simulink model "GeneralFEVmodel"  (R2022a)
settings: Solver=ode4  StartTime=0  StopTime=endtime  MaxStep=0.05  RelTol=1e-5
values from neighbouring files (symbols this model uses):
  EtaEM = Eta    [CreateEMmapII.m]
  Pbatt_max_new = 150*Mbatt    [CreateBATTmap.m]
  PtoTem = zeros(length(Pem),4)    [CreateEMmapII.m]
  Tem = Tem_max.*Tref/max(Tref)    [CreateEMmapII.m]
  Tem_lim = min([Tem_max*ones(1,length(Wem)); Pem_max./Wem])    [CreateEMmapII.m]
  Wem = wem_max.*w/max(w)    [CreateEMmapII.m]
undefined symbols (not defined in the file or in its folder): Av, Cd, Cr, EtaBATT, EtaGEAR, EtaPE, grav, Mv, Number_of_gears, Paux, Pbatt, Pem_max, rho_air, rw, SOC_batt_start_value, SOC_tract_max, SOC_tract_min, Tem_max, utvx_max, Utvx_vect, Wbatt, wem_max, wem_min
libraries: simulink_need_slupdate x1, simulink x1
settings Model: ExtModeTrigMode=oneshot  ExtModeArmWhenConnect=off  Creator=Mats  LastModifiedBy=Albin
settings SolverCC: AlgebraicLoopSolver=TrustRegion
settings DataIOCC: SaveFormat=Array  SignalLoggingSaveFormat=ModelDataLogs  ReturnWorkspaceOutputs=off  SignalLoggingName=sigsOut
settings OptimizationCC: BlockReduction=off  BooleanDataType=off  DefaultParameterBehavior=Inlined  BufferReuse=off  ExpressionDepthLimit=2147483647  InitFltsAndDblsToZero=on  LifeSpan=inf
settings DebuggingCC: ConsistencyChecking=warning  SaveWithParameterizedLinksMsg=none  UnderspecifiedInitializationDetection=Classic  MergeDetectMultiDrivingBlocksExec=none  SignalResolutionControl=TryResolveAllWithWarning  MultiTaskDSMMsg=warning  MultiTaskCondExecSysMsg=none  UnnecessaryDatatypeConvMsg=warning  FcnCallInpInsideContextMsg=warning  StateNameClashWarn=warning  SFUnexpectedBacktrackingDiag=warning  SFNoUnconditionalDefaultTransitionDiag=warning  SFMachineParentedDataDiag=warning  ArithmeticOperatorsInVariantConditions=warning
settings HardwareCC: ProdBitPerPointer=32  ProdBitPerSizeT=32  ProdBitPerPtrDiffT=32  ProdLargestAtomicFloat=None  ProdIntDivRoundTo=Undefined  ProdEndianess=Unspecified  ProdWordSize=32  ProdHWDeviceType=32-bit Generic  TargetHWDeviceType=32-bit Generic  TargetUnknown=on  ProdEqTarget=off
settings ModelReferenceCC: PropagateSignalLabelsOutOfModel=off
settings SFSimCC: SimUseLocalCustomCode=off  CustomCodeUndefinedFunction=UseInterfaceOnly
settings RTWCC: RTWUseLocalCustomCode=off  DLArmComputeVersion=19.05
settings CodeAppCC: StateflowObjectComments=on
settings GRTTargetCC: TargetFcnLib=ansi_tfl_tmw.mat  TargetLangStandard=C89/C90 (ANSI)  CombineOutputUpdateFcns=off  GRTInterface=on
settings ConfigComp: CovMetricSettings=dw  CovSaveCumulativeToWorkspaceVar=on  CovSaveSingleToWorkspaceVar=on  CovExternalEMLEnable=off

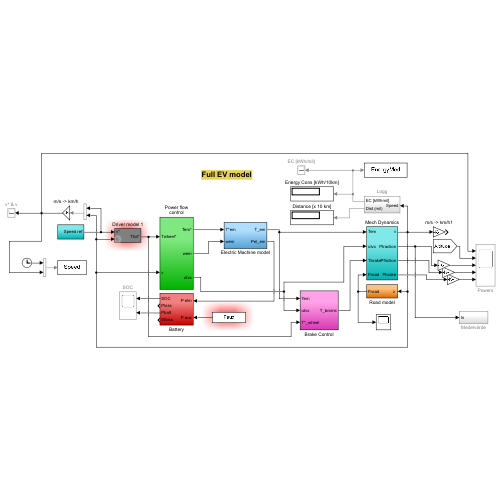
[thumbnail: Simulink's stored preview of the top-level diagram]
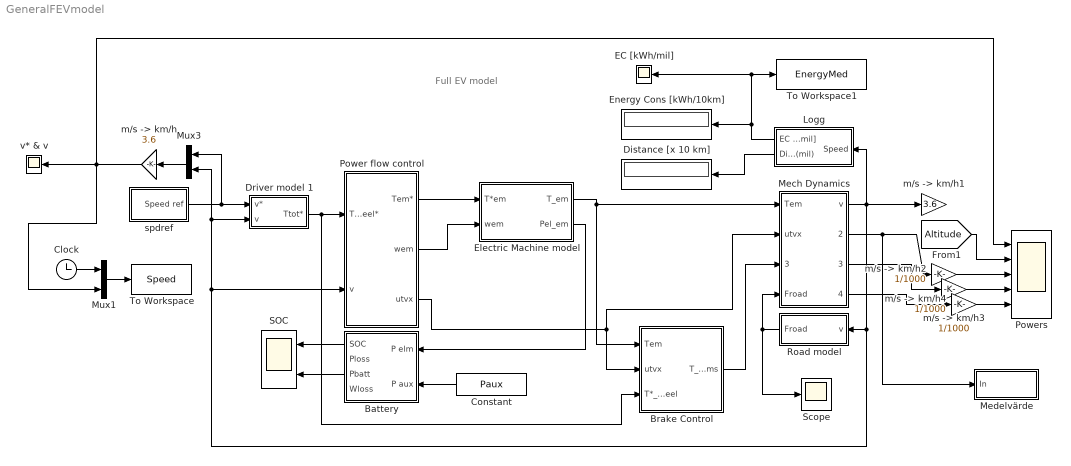
== system GeneralFEVmodel ==
  note: Full EV model
  Battery : Subsystem
  Brake Control : Subsystem
  Clock : Clock
  Constant : Constant  Value=Paux
  Distance [x 10 km] : Display
  Driver model 1 : Subsystem  mask{Mv=Mv, rw=rw, Pmax=Pem_max}
      mask prompts: Mv "Vehicle Mass"; rw "Wheel Radius"; Pmax "Max Wheel Power"
      mask init:
      | Ti = 2 + 1*(Mv-1000)/19000;
      | Kv=4*Mv/Ti;
  EC [kWh/mil] : Scope
  Electric Machine model : Subsystem
  Energy Cons [kWh/10km] : Display
  Logg : Subsystem
  Mech Dynamics : Subsystem
  Medelvärde : Subsystem
  Mux1 : Mux  Inputs=2
  Mux3 : Mux  Inputs=2
  Power flow control : Subsystem
  Powers : Scope  NumInputPorts=5
  Road model : Subsystem
  SOC : Scope  NumInputPorts=2
  Scope : Scope
  To Workspace : ToWorkspace  VariableName=Speed  SampleTime=-1
  To Workspace1 : ToWorkspace  VariableName=EnergyMed  SaveFormat=Timeseries  SampleTime=-1
  "m/s -> km/h" : Gain  Gain=3.6  SaturateOnIntegerOverflow=on  OutDataTypeStr=Inherit: Same as input  ParamDataTypeStr=Inherit: Same as input
  "m/s -> km/h1" : Gain  Gain=3.6  SaturateOnIntegerOverflow=on  OutDataTypeStr=Inherit: Same as input  ParamDataTypeStr=Inherit: Same as input
  "m/s -> km/h2" : Gain  Gain=1/1000  SaturateOnIntegerOverflow=on  OutDataTypeStr=Inherit: Same as input  ParamDataTypeStr=Inherit: Same as input
  "m/s -> km/h3" : Gain  Gain=1/1000  SaturateOnIntegerOverflow=on  OutDataTypeStr=Inherit: Same as input  ParamDataTypeStr=Inherit: Same as input
  "m/s -> km/h4" : Gain  Gain=1/1000  SaturateOnIntegerOverflow=on  OutDataTypeStr=Inherit: Same as input  ParamDataTypeStr=Inherit: Same as input
  spdref : Subsystem
  v* & v : Scope
  wires:
  Power flow control/2(wem) -> Electric Machine model/2(wem)
  Constant/1 -> Battery/2(P aux)
  spdref/1(Speed ref) -> Driver model 1/1(v*), Mux3/1
  Driver model 1/1(Ttot*) -> Brake Control/3(T*_wheel), Power flow control/1(Twheel*)
  Mux3/1 -> "m/s -> km/h"/1
  Power flow control/3(utvx) -> Brake Control/2(utvx), Mech Dynamics/2(utvx)
  Power flow control/1(Tem*) -> Electric Machine model/1(T*em)
  Mech Dynamics/1(v) -> Logg/1(Speed), Driver model 1/2(v), Mux3/2, Power flow control/2(v), Road model/1("v "), "m/s -> km/h1"/1
  Electric Machine model/1(T_em) -> Brake Control/1(Tem), Mech Dynamics/1(Tem)
  Electric Machine model/2(Pel_em) -> Battery/1(P elm)
  "m/s -> km/h"/1 -> Powers/1, Mux1/2, v* & v/1
  Battery/1(SOC) -> SOC/1
  Battery/3(Pbatt) -> SOC/2
  [Altitude] -> Powers/2
  Mech Dynamics/2(Ptraction) -> Medelvärde/1(In), "m/s -> km/h2"/1
  Mech Dynamics/3(Pfriction) -> "m/s -> km/h3"/1
  Mech Dynamics/4(Pbrake) -> "m/s -> km/h4"/1
  "m/s -> km/h2"/1 -> Powers/3
  "m/s -> km/h3"/1 -> Powers/4
  "m/s -> km/h4"/1 -> Powers/5
  Brake Control/1(T_broms) -> Mech Dynamics/3(Tbrake)
  Road model/1(Froad) -> Scope/1, Mech Dynamics/4(Froad)
  Clock/1 -> Mux1/1
  Mux1/1 -> To Workspace/1
  Logg/1(EC [kWhmil]) -> EC [kWh/mil]/1, To Workspace1/1, Energy Cons [kWh/10km]/1
  Logg/2(Dist (mil)) -> Distance [x 10 km]/1

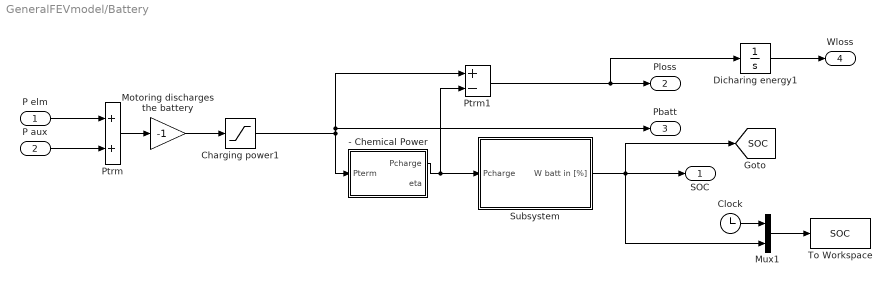
== system GeneralFEVmodel/Battery ==
  P elm : Inport
  P aux : Inport  Port=2
  - Chemical Power : Subsystem
  Charging power1 : Saturate  UpperLimit=Pbatt_max_new  LowerLimit=-Pbatt_max_new
  Clock : Clock
  Dicharing energy1 : Integrator  UpperSaturationLimit=-1
  Motoring discharges the battery : Gain  Gain=-1  SaturateOnIntegerOverflow=on  OutDataTypeStr=Inherit: Same as input  ParamDataTypeStr=Inherit: Same as input
  Mux1 : Mux  Inputs=2
  Ptrm : Sum  InputSameDT=on  SaturateOnIntegerOverflow=on  OutDataTypeStr=Inherit: Same as first input
  Ptrm1 : Sum  Inputs=+-  InputSameDT=on  SaturateOnIntegerOverflow=on  OutDataTypeStr=Inherit: Same as first input
  Subsystem : Subsystem
  To Workspace : ToWorkspace  VariableName=SOC  SampleTime=1
  SOC : Outport  InitialOutput=0  VectorParamsAs1DForOutWhenUnconnected=off
  Ploss : Outport  Port=2  InitialOutput=0  VectorParamsAs1DForOutWhenUnconnected=off
  Pbatt : Outport  Port=3  InitialOutput=0  VectorParamsAs1DForOutWhenUnconnected=off
  Wloss : Outport  Port=4  InitialOutput=0  VectorParamsAs1DForOutWhenUnconnected=off
  tag scope: SOC=global
  wires:
  P elm/1 -> Ptrm/1
  Ptrm/1 -> Motoring discharges the battery/1
  - Chemical Power/1(Pcharge) -> Ptrm1/2, Subsystem/1("Pcharge ")
  Ptrm1/1 -> Ploss/1, Dicharing energy1/1
  Motoring discharges the battery/1 -> Charging power1/1
  P aux/1 -> Ptrm/2
  Dicharing energy1/1 -> Wloss/1
  Charging power1/1 -> Pbatt/1, Ptrm1/1, - Chemical Power/1(Pterm)
  Subsystem/1(W batt in [%]) -> Mux1/2, SOC/1, [SOC]
  Clock/1 -> Mux1/1
  Mux1/1 -> To Workspace/1

== system GeneralFEVmodel/Brake Control ==
  note: If the drive train is not able
      | to supply the braking force, then
      | the friction brakes are used.
  Tem : Inport
  utvx : Inport  Port=2
  T*_wheel : Inport  Port=3
  -> hjulmoment : Product  InputSameDT=on  SaturateOnIntegerOverflow=on  OutDataTypeStr=Inherit: Same as first input
  Endast negativa bromsmoment1 : Saturate  UpperLimit=0  LowerLimit=-inf
  Sum1 : Sum  Inputs=-+  InputSameDT=on  SaturateOnIntegerOverflow=on  OutDataTypeStr=Inherit: Same as first input
  T_broms : Outport  InitialOutput=0  VectorParamsAs1DForOutWhenUnconnected=off
  wires:
  Tem/1 -> -> hjulmoment/1
  utvx/1 -> -> hjulmoment/2
  -> hjulmoment/1 -> Sum1/1
  T*_wheel/1 -> Sum1/2
  Sum1/1 -> Endast negativa bromsmoment1/1
  Endast negativa bromsmoment1/1 -> T_broms/1

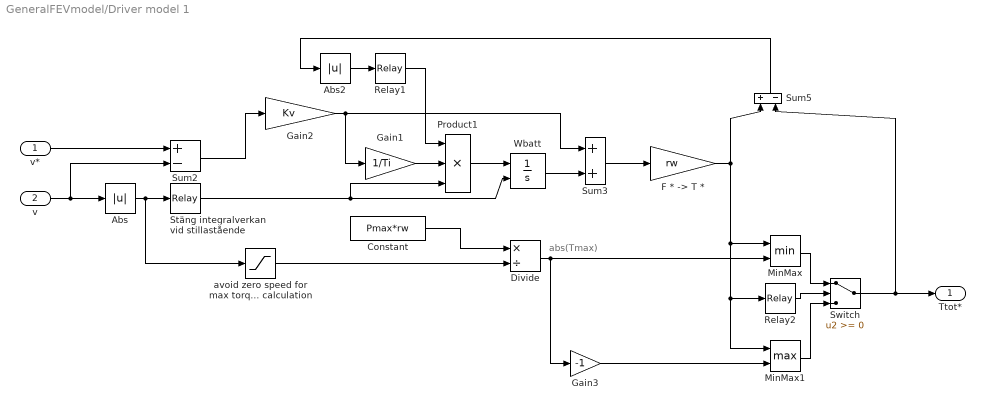
== system GeneralFEVmodel/Driver model 1 ==
  note: abs(Tmax)
  v* : Inport
  v : Inport  Port=2
  Abs : Abs
  Abs2 : Abs
  Constant : Constant  Value=Pmax*rw
  Divide : Product  Inputs=*/
  "F * -> T *" : Gain  Gain=rw  SaturateOnIntegerOverflow=on  OutDataTypeStr=Inherit: Same as input  ParamDataTypeStr=Inherit: Same as input
  Gain1 : Gain  Gain=1/Ti  SaturateOnIntegerOverflow=on  OutDataTypeStr=Inherit: Same as input  ParamDataTypeStr=Inherit: Same as input
  Gain2 : Gain  Gain=Kv  SaturateOnIntegerOverflow=on  OutDataTypeStr=Inherit: Same as input  ParamDataTypeStr=Inherit: Same as input
  Gain3 : Gain  Gain=-1  SaturateOnIntegerOverflow=on  OutDataTypeStr=Inherit: Same as input  ParamDataTypeStr=Inherit: Same as input
  MinMax : MinMax  Inputs=2
  MinMax1 : MinMax  Function=max  Inputs=2
  Product1 : Product  Inputs=3  InputSameDT=on  SaturateOnIntegerOverflow=on  OutDataTypeStr=Inherit: Same as first input
  Relay1 : Relay  OnOutputValue=0  OffOutputValue=1
  Relay2 : Relay  OnOutputValue=10  OffOutputValue=1
  Stäng integralverkan vid stillastående : Relay  OnSwitchValue=0.3  OffSwitchValue=0.3-eps
  Sum2 : Sum  Inputs=+-  InputSameDT=on  SaturateOnIntegerOverflow=on  OutDataTypeStr=Inherit: Same as first input
  Sum3 : Sum  InputSameDT=on  SaturateOnIntegerOverflow=on  OutDataTypeStr=Inherit: Same as first input
  Sum5 : Sum  Inputs=+-  InputSameDT=on  SaturateOnIntegerOverflow=on  OutDataTypeStr=Inherit: Same as first input
  Switch : Switch  SaturateOnIntegerOverflow=off  InputSameDT=off
  Wbatt : Integrator  ExternalReset=falling  LimitOutput=on  UpperSaturationLimit=15000  LowerSaturationLimit=-15000
  avoid zero speed for max torque calculation : Saturate  UpperLimit=inf  LowerLimit=5/3.6
  Ttot* : Outport  InitialOutput=0  VectorParamsAs1DForOutWhenUnconnected=off
  wires:
  Sum5/1 -> Abs2/1
  Relay1/1 -> Product1/1
  Abs2/1 -> Relay1/1
  Gain1/1 -> Product1/2
  Abs/1 -> Stäng integralverkan vid stillastående/1, avoid zero speed for max torque calculation/1
  Product1/1 -> Wbatt/1
  Sum3/1 -> "F * -> T *"/1
  Wbatt/1 -> Sum3/2
  "F * -> T *"/1 -> Sum5/1, MinMax/1, MinMax1/1, Relay2/1
  Gain2/1 -> Gain1/1, Sum3/1
  Stäng integralverkan vid stillastående/1 -> Product1/3, Wbatt/2
  Sum2/1 -> Gain2/1
  v*/1 -> Sum2/1
  v/1 -> Abs/1, Sum2/2
  Constant/1 -> Divide/1
  avoid zero speed for max torque calculation/1 -> Divide/2
  Divide/1 -> Gain3/1, MinMax/2
  Gain3/1 -> MinMax1/2
  Relay2/1 -> Switch/2
  MinMax/1 -> Switch/1
  MinMax1/1 -> Switch/3
  Switch/1 -> Ttot*/1, Sum5/2

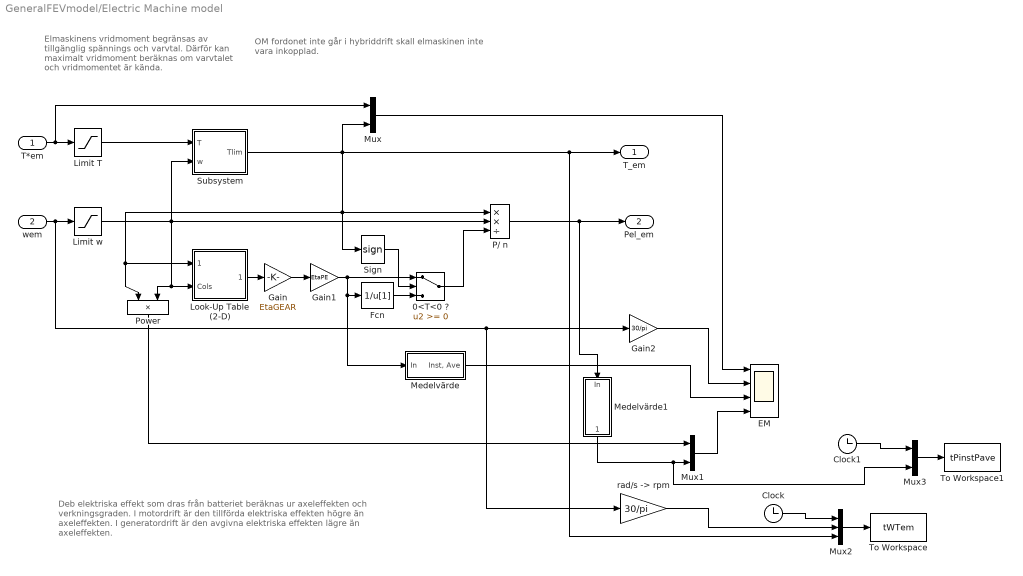
== system GeneralFEVmodel/Electric Machine model ==
  note: Elmaskinens vridmoment begränsas
      | av tillgänglig spännings och varvtal. Därför
      | kan maximalt vridmoment beräknas
      | om varvtalet och vridmomentet är kända.
  note: OM fordonet inte går i hybriddrift skall elmaskinen inte
      | vara inkopplad.
  note: Deb elektriska effekt som dras från batteriet beräknas ur axeleffekten
      | och verkningsgraden. I motordrift är den tillförda elektriska effekten
      | högre än axeleffekten. I generatordrift är den avgivna elektriska effekten
      | lägre än axeleffekten.
  T*em : Inport
  wem : Inport  Port=2
  0<T<0 ? : Switch
  Clock : Clock
  Clock1 : Clock
  EM : Scope  NumInputPorts=4
  Fcn : Fcn  Expr=1/u[1]
  Gain : Gain  Gain=EtaGEAR  SaturateOnIntegerOverflow=on  OutDataTypeStr=Inherit: Same as input  ParamDataTypeStr=Inherit: Same as input
  Gain1 : Gain  Gain=EtaPE  SaturateOnIntegerOverflow=on  OutDataTypeStr=Inherit: Same as input  ParamDataTypeStr=Inherit: Same as input
  Gain2 : Gain  Gain=30/pi  SaturateOnIntegerOverflow=on  OutDataTypeStr=Inherit: Same as input  ParamDataTypeStr=Inherit: Same as input
  Limit T : Saturate  UpperLimit=Tem_max  LowerLimit=-Tem_max
  Limit w : Saturate  UpperLimit=wem_max  LowerLimit=0
  Look-Up Table (2-D) : Subsystem  mask(Lookup Table (2-D)){x=Tem, y=Wem, t=EtaEM}
      mask prompts: x "Row:"; y "Column:"; t "Table:"
      mask help: Performs 2-D linear interpolation of input values using the specified input/output table. Extrapolation is performed outside the table boundaries. The first dimension corresponds to the top (or left) input port.
      mask init:
      | [r,c]=size(t);
      | xt=reshape(x,prod(size(x)),1);
      | xi=xt(:,ones(1,c));
      | minx=min(x); maxx=max(x);
      | mint=min(min(t)); maxt=max(max(t));
      mask Display: plot(double(xi),double(t),double([minx maxx]),double([mint mint]),double([minx minx]),double([mint maxt]))
  Medelvärde : Subsystem
  Medelvärde1 : Subsystem
  Mux : Mux  Inputs=2
  Mux1 : Mux  Inputs=2
  Mux2 : Mux  Inputs=3
  Mux3 : Mux  Inputs=2
  P/ n : Product  Inputs=**/  InputSameDT=on  SaturateOnIntegerOverflow=on  OutDataTypeStr=Inherit: Same as first input
  Power : Product  SaturateOnIntegerOverflow=on  OutDataTypeStr=Inherit: Same as first input
  Sign : Signum
  Subsystem : Subsystem  mask{Tmax=Tem_max, Pmax=Pem_max}
      mask prompts: Tmax "Max Torque"; Pmax "Max Power"
      mask Display:
      | plot(-120,-120,120,120)
      | plot([-110 110],[0 0],[0 0],[-110 110])
      | plot([-20 20],[90 90],[-20 20],[-90 -90])
      | 
      | plot([-100 :-20],-90*20./[-100:-20])
      | plot([-100 :-20],90*20./[-100:-20])
      | plot([20:100],-90*20./[20:100])
      | plot([20:100],90*20./[20:100])
  To Workspace : ToWorkspace  VariableName=tWTem  SampleTime=-1
  To Workspace1 : ToWorkspace  VariableName=tPinstPave  SampleTime=-1
  "rad/s -> rpm" : Gain  Gain=30/pi  SaturateOnIntegerOverflow=on  OutDataTypeStr=Inherit: Same as input  ParamDataTypeStr=Inherit: Same as input
  T_em : Outport  InitialOutput=0  VectorParamsAs1DForOutWhenUnconnected=off
  Pel_em : Outport  Port=2  InitialOutput=0  VectorParamsAs1DForOutWhenUnconnected=off
  wires:
  wem/1 -> Limit w/1, Gain2/1, "rad/s -> rpm"/1
  Sign/1 -> 0<T<0 ?/2
  P/ n/1 -> Medelvärde1/1(In), Pel_em/1
  T*em/1 -> Limit T/1, Mux/1
  Fcn/1 -> 0<T<0 ?/3
  Look-Up Table (2-D)/1(Out1) -> Gain/1
  Limit T/1 -> Subsystem/1(T)
  Limit w/1 -> Look-Up Table (2-D)/2(Cols), Power/2, P/ n/2, Subsystem/2(w)
  Medelvärde/1("Inst, Ave") -> EM/3
  Mux/1 -> EM/1
  Power/1 -> Mux1/1
  Mux1/1 -> EM/4
  Gain/1 -> Gain1/1
  Gain1/1 -> 0<T<0 ?/1, Medelvärde/1(In), Fcn/1
  Subsystem/1(Tlim) -> Mux/2, Power/1, Look-Up Table (2-D)/1(Rows), Sign/1, P/ n/1, T_em/1, Mux2/3
  0<T<0 ?/1 -> P/ n/3
  "rad/s -> rpm"/1 -> Mux2/2
  Clock/1 -> Mux2/1
  Mux2/1 -> To Workspace/1
  Gain2/1 -> EM/2
  Medelvärde1/1("Inst, Ave") -> Mux3/2, Mux1/2
  Clock1/1 -> Mux3/1
  Mux3/1 -> To Workspace1/1

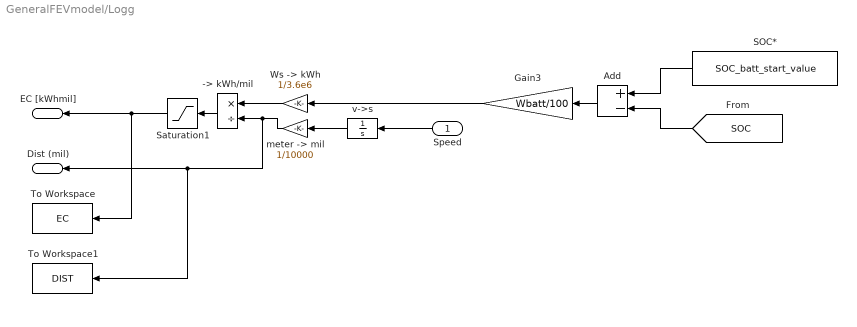
== system GeneralFEVmodel/Logg ==
  Speed : Inport
  -> kWh/mil : Product  Inputs=*/  InputSameDT=on  SaturateOnIntegerOverflow=on  OutDataTypeStr=Inherit: Same as first input
  Add : Sum  Inputs=+-
  Gain3 : Gain  Gain=Wbatt/100  SaturateOnIntegerOverflow=on  OutDataTypeStr=Inherit: Same as input  ParamDataTypeStr=Inherit: Same as input
  SOC* : Constant  Value=SOC_batt_start_value
  Saturation1 : Saturate  UpperLimit=inf  LowerLimit=eps
  To Workspace : ToWorkspace  VariableName=EC  SampleTime=-1
  To Workspace1 : ToWorkspace  VariableName=DIST  SampleTime=-1
  "Ws -> kWh" : Gain  Gain=1/3.6e6  SaturateOnIntegerOverflow=on  OutDataTypeStr=Inherit: Same as input  ParamDataTypeStr=Inherit: Same as input
  "meter -> mil" : Gain  Gain=1/10000  SaturateOnIntegerOverflow=on  OutDataTypeStr=Inherit: Same as input  ParamDataTypeStr=Inherit: Same as input
  v->s : Integrator  InitialCondition=100  LimitOutput=on  LowerSaturationLimit=100
  EC [kWhmil] : Outport  VectorParamsAs1DForOutWhenUnconnected=off
  Dist (mil) : Outport  Port=2  VectorParamsAs1DForOutWhenUnconnected=off
  wires:
  "Ws -> kWh"/1 -> -> kWh/mil/1
  v->s/1 -> "meter -> mil"/1
  -> kWh/mil/1 -> Saturation1/1
  Speed/1 -> v->s/1
  Saturation1/1 -> EC [kWhmil]/1, To Workspace/1
  "meter -> mil"/1 -> -> kWh/mil/2, To Workspace1/1, Dist (mil)/1
  SOC*/1 -> Add/1
  [SOC] -> Add/2
  Add/1 -> Gain3/1
  Gain3/1 -> "Ws -> kWh"/1

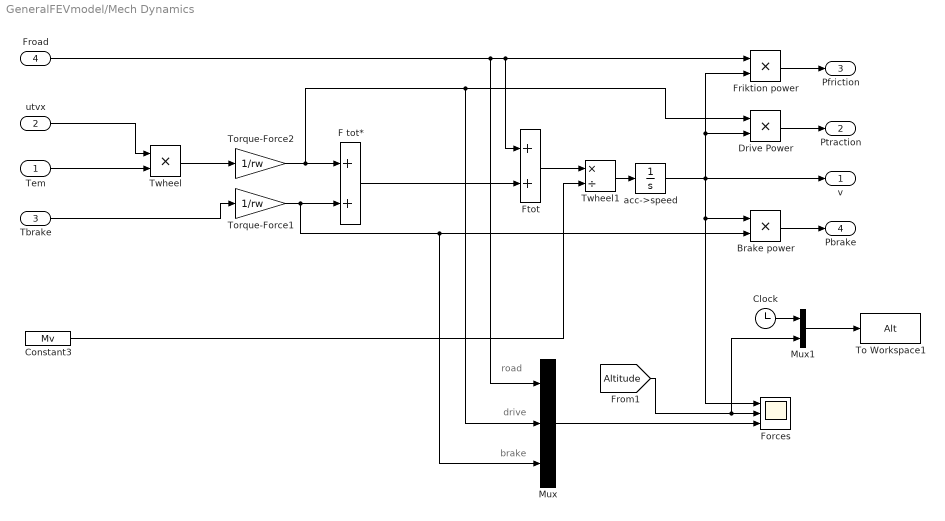
== system GeneralFEVmodel/Mech Dynamics ==
  note: road
  note: drive
  note: brake
  Tem : Inport
  utvx : Inport  Port=2
  Tbrake : Inport  Port=3
  Froad : Inport  Port=4
  Brake power : Product  InputSameDT=on  SaturateOnIntegerOverflow=on  OutDataTypeStr=Inherit: Same as first input
  Clock : Clock
  Constant3 : Constant  Value=Mv
  Drive Power : Product  InputSameDT=on  SaturateOnIntegerOverflow=on  OutDataTypeStr=Inherit: Same as first input
  F tot* : Sum  InputSameDT=on  SaturateOnIntegerOverflow=on  OutDataTypeStr=Inherit: Same as first input
  Forces : Scope  NumInputPorts=3
  Friktion power : Product  InputSameDT=on  SaturateOnIntegerOverflow=on  OutDataTypeStr=Inherit: Same as first input
  Ftot : Sum  InputSameDT=on  SaturateOnIntegerOverflow=on  OutDataTypeStr=Inherit: Same as first input
  Mux : Mux  Inputs=3
  Mux1 : Mux  Inputs=2
  To Workspace1 : ToWorkspace  VariableName=Alt  SampleTime=-1
  Torque-Force1 : Gain  Gain=1/rw  SaturateOnIntegerOverflow=on  OutDataTypeStr=Inherit: Same as input  ParamDataTypeStr=Inherit: Same as input
  Torque-Force2 : Gain  Gain=1/rw  SaturateOnIntegerOverflow=on  OutDataTypeStr=Inherit: Same as input  ParamDataTypeStr=Inherit: Same as input
  Twheel : Product  InputSameDT=on  SaturateOnIntegerOverflow=on  OutDataTypeStr=Inherit: Same as first input
  Twheel1 : Product  Inputs=*/  InputSameDT=on  SaturateOnIntegerOverflow=on  OutDataTypeStr=Inherit: Same as first input
  acc->speed : Integrator  LimitOutput=on  LowerSaturationLimit=0
  v : Outport  InitialOutput=0  VectorParamsAs1DForOutWhenUnconnected=off
  Ptraction : Outport  Port=2  InitialOutput=0  VectorParamsAs1DForOutWhenUnconnected=off
  Pfriction : Outport  Port=3  InitialOutput=0  VectorParamsAs1DForOutWhenUnconnected=off
  Pbrake : Outport  Port=4  InitialOutput=0  VectorParamsAs1DForOutWhenUnconnected=off
  wires:
  Twheel1/1 -> acc->speed/1
  acc->speed/1 -> Friktion power/2, Drive Power/2, Brake power/1, Forces/1, v/1
  Tbrake/1 -> Torque-Force1/1
  F tot*/1 -> Ftot/2
  Ftot/1 -> Twheel1/1
  Froad/1 -> Ftot/1, Friktion power/1, Mux/1
  Friktion power/1 -> Pfriction/1
  Constant3/1 -> Twheel1/2
  [Altitude] -> Mux1/2, Forces/2
  Mux/1 -> Forces/3
  Drive Power/1 -> Ptraction/1
  Torque-Force1/1 -> F tot*/2, Brake power/2, Mux/3
  Torque-Force2/1 -> Drive Power/1, Mux/2, F tot*/1
  Brake power/1 -> Pbrake/1
  Twheel/1 -> Torque-Force2/1
  utvx/1 -> Twheel/1
  Tem/1 -> Twheel/2
  Clock/1 -> Mux1/1
  Mux1/1 -> To Workspace1/1

== system GeneralFEVmodel/Medelvärde ==
  note: Denna del "mäter" tiden då motorn
      | är till, d.v.s. då verkningsgraden är
      | större än 1 %. Om den är 5 % antas
      | motorn stå still.
  In : Inport
  Integral : Integrator
  Integral1 : Integrator  InitialCondition=eps  LimitOutput=on  LowerSaturationLimit=eps
  Medelv : Product  Inputs=*/  InputSameDT=on  SaturateOnIntegerOverflow=on  OutDataTypeStr=Inherit: Same as first input
  Medelv1 : Product  Inputs=**  InputSameDT=on  SaturateOnIntegerOverflow=on  OutDataTypeStr=Inherit: Same as first input
  Mux : Mux  Inputs=2
  Relay : Relay  OnSwitchValue=0.05  OffSwitchValue=0.04
  Scope : Scope
  wires:
  Mux/1 -> Scope/1
  Medelv/1 -> Mux/2
  Relay/1 -> Integral1/1, Medelv1/2
  In/1 -> Relay/1, Medelv1/1, Mux/1
  Integral/1 -> Medelv/1
  Integral1/1 -> Medelv/2
  Medelv1/1 -> Integral/1

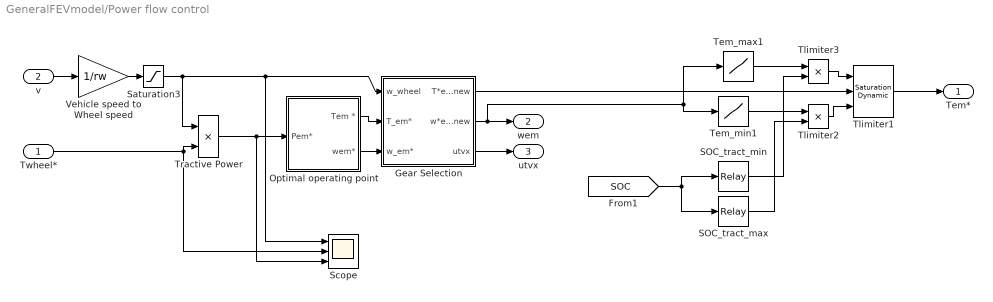
== system GeneralFEVmodel/Power flow control ==
  Twheel* : Inport
  v : Inport  Port=2
  Gear Selection : Subsystem
  Optimal operating point : Subsystem
  SOC_tract_max : Relay  OnSwitchValue=SOC_tract_max+1  OffSwitchValue=SOC_tract_max-1  OnOutputValue=0  OffOutputValue=1
  SOC_tract_min : Relay  OnSwitchValue=SOC_tract_min+1  OffSwitchValue=SOC_tract_min-1
  Saturation3 : Saturate  UpperLimit=inf  LowerLimit=1
  Scope : Scope  NumInputPorts=3
  Tem_max1 : Lookup  InputValues=Wem  Table=Tem_lim
  Tem_min1 : Lookup  InputValues=Wem  Table=-Tem_lim
  Tlimiter1 : simulink/Discontinuities/Saturation Dynamic  OutMin=[]  OutMax=[]  OutDataTypeStr=Inherit: Same as second input  OutDataType=fixdt(1, 16)  OutScaling=2^-10  DoSatur=off
  Tlimiter2 : Product  Inputs=**  InputSameDT=on  SaturateOnIntegerOverflow=on  OutDataTypeStr=Inherit: Same as first input
  Tlimiter3 : Product  Inputs=**  InputSameDT=on  SaturateOnIntegerOverflow=on  OutDataTypeStr=Inherit: Same as first input
  Tractive Power : Product  InputSameDT=on  SaturateOnIntegerOverflow=on  OutDataTypeStr=Inherit: Same as first input
  Vehicle speed to Wheel speed : Gain  Gain=1/rw  SaturateOnIntegerOverflow=on  OutDataTypeStr=Inherit: Same as input  ParamDataTypeStr=Inherit: Same as input
  Tem* : Outport  VectorParamsAs1DForOutWhenUnconnected=off
  wem : Outport  Port=2  VectorParamsAs1DForOutWhenUnconnected=off
  utvx : Outport  Port=3  VectorParamsAs1DForOutWhenUnconnected=off
  wires:
  Vehicle speed to Wheel speed/1 -> Saturation3/1
  Twheel*/1 -> Tractive Power/2, Scope/2
  v/1 -> Vehicle speed to Wheel speed/1
  Gear Selection/3(utvx) -> utvx/1
  Optimal operating point/2(wem*) -> Gear Selection/3(w_em*)
  Optimal operating point/1(Tem *) -> Gear Selection/2(T_em*)
  Tractive Power/1 -> Scope/3, Optimal operating point/1(Pem*)
  Gear Selection/1(T*em_new) -> Tlimiter1/2
  Gear Selection/2(w*em_new) -> wem/1, Tem_max1/1, Tem_min1/1
  [SOC] -> SOC_tract_max/1, SOC_tract_min/1
  Tem_max1/1 -> Tlimiter3/1
  Tlimiter3/1 -> Tlimiter1/1
  Tem_min1/1 -> Tlimiter2/1
  Tlimiter2/1 -> Tlimiter1/3
  SOC_tract_min/1 -> Tlimiter3/2
  SOC_tract_max/1 -> Tlimiter2/2
  Tlimiter1/1 -> Tem*/1
  Saturation3/1 -> Tractive Power/1, Scope/1, Gear Selection/1(w_wheel)

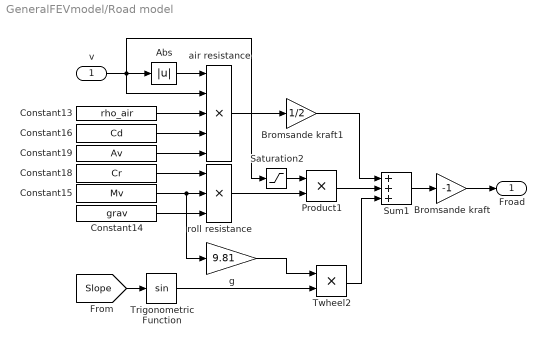
== system GeneralFEVmodel/Road model ==
  "v " : Inport
  Abs : Abs
  Bromsande kraft : Gain  Gain=-1  SaturateOnIntegerOverflow=on  OutDataTypeStr=Inherit: Same as input  ParamDataTypeStr=Inherit: Same as input
  Bromsande kraft1 : Gain  Gain=1/2  SaturateOnIntegerOverflow=on  OutDataTypeStr=Inherit: Same as input  ParamDataTypeStr=Inherit: Same as input
  Constant13 : Constant  Value=rho_air
  Constant14 : Constant  Value=grav
  Constant15 : Constant  Value=Mv
  Constant16 : Constant  Value=Cd
  Constant18 : Constant  Value=Cr
  Constant19 : Constant  Value=Av
  Product1 : Product  InputSameDT=on  SaturateOnIntegerOverflow=on  OutDataTypeStr=Inherit: Same as first input
  Saturation2 : Saturate  UpperLimit=1  LowerLimit=-1
  Sum1 : Sum  Inputs=+++  InputSameDT=on  SaturateOnIntegerOverflow=on  OutDataTypeStr=Inherit: Same as first input
  Trigonometric Function : Trigonometry
  Twheel2 : Product  Inputs=**  InputSameDT=on  SaturateOnIntegerOverflow=on  OutDataTypeStr=Inherit: Same as first input
  air resistance : Product  Inputs=5  InputSameDT=on  SaturateOnIntegerOverflow=on  OutDataTypeStr=Inherit: Same as first input
  g : Gain  Gain=9.81  SaturateOnIntegerOverflow=on  OutDataTypeStr=Inherit: Same as input  ParamDataTypeStr=Inherit: Same as input
  roll resistance : Product  Inputs=3  InputSameDT=on  SaturateOnIntegerOverflow=on  OutDataTypeStr=Inherit: Same as first input
  Froad : Outport  InitialOutput=0  VectorParamsAs1DForOutWhenUnconnected=off
  wires:
  Abs/1 -> air resistance/1
  Constant18/1 -> roll resistance/1
  Constant19/1 -> air resistance/5
  Constant16/1 -> air resistance/4
  Constant13/1 -> air resistance/3
  Constant14/1 -> roll resistance/3
  Product1/1 -> Sum1/2
  air resistance/1 -> Bromsande kraft1/1
  Saturation2/1 -> Product1/1
  roll resistance/1 -> Product1/2
  Sum1/1 -> Bromsande kraft/1
  "v "/1 -> Abs/1, Saturation2/1, air resistance/2
  Bromsande kraft/1 -> Froad/1
  Bromsande kraft1/1 -> Sum1/1
  Trigonometric Function/1 -> Twheel2/2
  Constant15/1 -> g/1, roll resistance/2
  [Slope] -> Trigonometric Function/1
  Twheel2/1 -> Sum1/3
  g/1 -> Twheel2/1

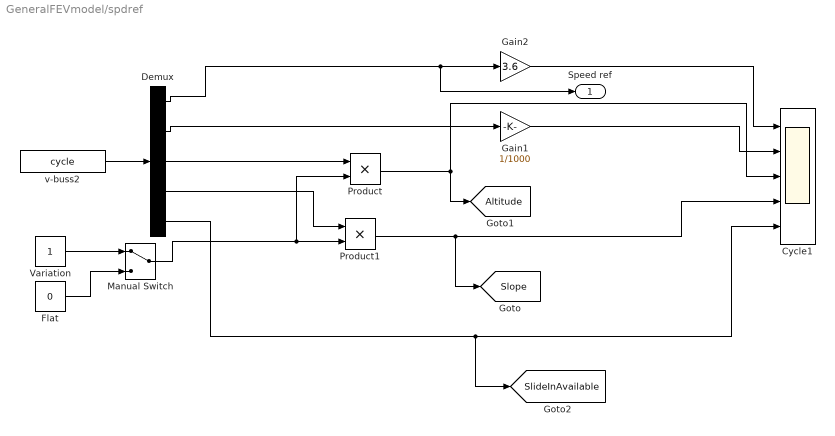
== system GeneralFEVmodel/spdref ==
  Cycle1 : Scope  NumInputPorts=5
  Demux : Demux  Outputs=5
  Flat : Constant  Value=0
  Gain1 : Gain  Gain=1/1000  SaturateOnIntegerOverflow=on  OutDataTypeStr=Inherit: Same as input  ParamDataTypeStr=Inherit: Same as input
  Gain2 : Gain  Gain=3.6  SaturateOnIntegerOverflow=on  OutDataTypeStr=Inherit: Same as input  ParamDataTypeStr=Inherit: Same as input
  Manual Switch : ManualSwitch
  Product : Product
  Product1 : Product
  Variation : Constant
  v-buss2 : FromWorkspace  VariableName=cycle  SampleTime=.2  ZeroCross=off
  Speed ref : Outport  VectorParamsAs1DForOutWhenUnconnected=off
  tag scope: Altitude=global, SlideInAvailable=global, Slope=global
  wires:
  v-buss2/1 -> Demux/1
  Demux/2 -> Gain1/1
  Flat/1 -> Manual Switch/2
  Product/1 -> Cycle1/3, [Altitude]
  Product1/1 -> Cycle1/4, [Slope]
  Variation/1 -> Manual Switch/1
  Manual Switch/1 -> Product/2, Product1/2
  Gain1/1 -> Cycle1/2
  Gain2/1 -> Cycle1/1
  Demux/5 -> Cycle1/5, [SlideInAvailable]
  Demux/3 -> Product/1
  Demux/4 -> Product1/1
  Demux/1 -> Speed ref/1, Gain2/1

== system GeneralFEVmodel/Battery/- Chemical Power ==
  Pterm : Inport
  Look-Up Table : Lookup  InputValues=Pbatt  Table=EtaBATT
  P/ n : Product  Inputs=**  InputSameDT=on  SaturateOnIntegerOverflow=on  OutDataTypeStr=Inherit: Same as first input
  Saturation : Saturate  UpperLimit=max(Pbatt)  LowerLimit=min(Pbatt)
  Pcharge : Outport  InitialOutput=0  VectorParamsAs1DForOutWhenUnconnected=off
  eta : Outport  Port=2  InitialOutput=0  VectorParamsAs1DForOutWhenUnconnected=off
  wires:
  Pterm/1 -> P/ n/1, Saturation/1
  Saturation/1 -> Look-Up Table/1
  P/ n/1 -> Pcharge/1
  Look-Up Table/1 -> P/ n/2, eta/1

== system GeneralFEVmodel/Battery/Subsystem ==
  "Pcharge " : Inport
  Gain3 : Gain  Gain=100/Wbatt  SaturateOnIntegerOverflow=on  OutDataTypeStr=Inherit: Same as input  ParamDataTypeStr=Inherit: Same as input
  Saturation : Saturate  UpperLimit=100  LowerLimit=0
  W batt starts at 70% : Integrator  InitialCondition=SOC_batt_start_value/100*Wbatt  LimitOutput=on  UpperSaturationLimit=1.2*Wbatt  LowerSaturationLimit=0
  W batt in [%] : Outport  VectorParamsAs1DForOutWhenUnconnected=off
  wires:
  Gain3/1 -> Saturation/1
  W batt starts at 70%/1 -> Gain3/1
  Saturation/1 -> W batt in [%]/1
  "Pcharge "/1 -> W batt starts at 70%/1

== system GeneralFEVmodel/Electric Machine model/Look-Up Table (2-D) ==
  Rows : Inport
  Cols : Inport  Port=2
  Look-Up Table (2-D) : Lookup2D  RowIndex=x  ColumnIndex=y  Table=t
  Out1 : Outport  VectorParamsAs1DForOutWhenUnconnected=off
  wires:
  Rows/1 -> Look-Up Table (2-D)/1
  Cols/1 -> Look-Up Table (2-D)/2
  Look-Up Table (2-D)/1 -> Out1/1

== system GeneralFEVmodel/Electric Machine model/Medelvärde ==
  note: Denna del "mäter" tiden då motorn
      | är till, d.v.s. då verkningsgraden är
      | större än 1 %. Om den är 5 % antas
      | motorn stå still.
  In : Inport
  Integral : Integrator
  Integral1 : Integrator  InitialCondition=eps  LimitOutput=on  LowerSaturationLimit=eps
  Medelv : Product  Inputs=*/  InputSameDT=on  SaturateOnIntegerOverflow=on  OutDataTypeStr=Inherit: Same as first input
  Medelv1 : Product  Inputs=**  InputSameDT=on  SaturateOnIntegerOverflow=on  OutDataTypeStr=Inherit: Same as first input
  Mux : Mux  Inputs=2
  Relay : Relay  OnSwitchValue=0.05  OffSwitchValue=0.04
  "Inst, Ave" : Outport  VectorParamsAs1DForOutWhenUnconnected=off
  wires:
  Integral1/1 -> Medelv/2
  Integral/1 -> Medelv/1
  In/1 -> Relay/1, Mux/1, Medelv1/1
  Relay/1 -> Integral1/1, Medelv1/2
  Medelv/1 -> Mux/2
  Mux/1 -> "Inst, Ave"/1
  Medelv1/1 -> Integral/1

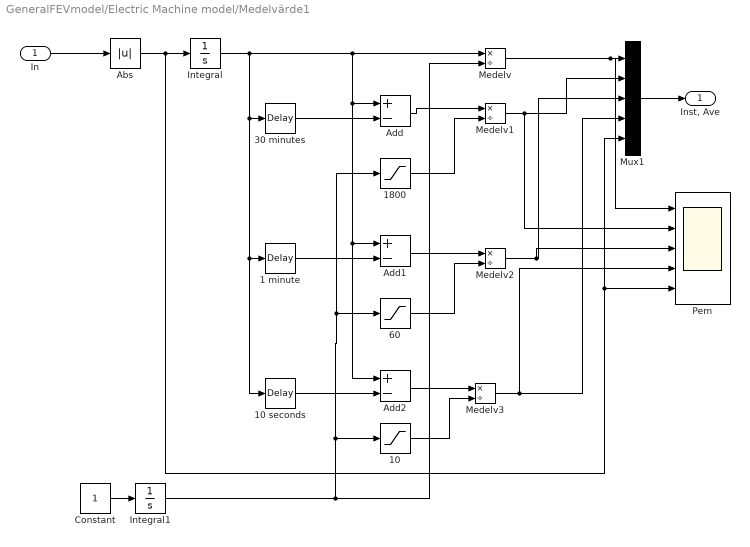
== system GeneralFEVmodel/Electric Machine model/Medelvärde1 ==
  In : Inport
  1 minute : TransportDelay  DelayTime=60
  10 : Saturate  UpperLimit=10  LowerLimit=0
  10 seconds : TransportDelay  DelayTime=10
  1800 : Saturate  UpperLimit=1800  LowerLimit=0
  30 minutes : TransportDelay  DelayTime=1800  BufferSize=18432
  60 : Saturate  UpperLimit=60  LowerLimit=0
  Abs : Abs  SaturateOnIntegerOverflow=off
  Add : Sum  Inputs=+-
  Add1 : Sum  Inputs=+-
  Add2 : Sum  Inputs=+-
  Constant : Constant
  Integral : Integrator
  Integral1 : Integrator  InitialCondition=eps  LimitOutput=on  LowerSaturationLimit=eps
  Medelv{,1..3} (4 alike) : Product  Inputs=*/  InputSameDT=on  SaturateOnIntegerOverflow=on  OutDataTypeStr=Inherit: Same as first input
  Mux1 : Mux  Inputs=5
  Pem : Scope  NumInputPorts=5
  "Inst, Ave" : Outport  VectorParamsAs1DForOutWhenUnconnected=off
  wires:
  In/1 -> Abs/1
  Integral1/1 -> Medelv/2, 1800/1, 60/1, 10/1
  Abs/1 -> Pem/5, Mux1/5, Integral/1
  Constant/1 -> Integral1/1
  30 minutes/1 -> Add/2
  Add/1 -> Medelv1/1
  1 minute/1 -> Add1/2
  10 seconds/1 -> Add2/2
  Add2/1 -> Medelv3/1
  Add1/1 -> Medelv2/1
  1800/1 -> Medelv1/2
  60/1 -> Medelv2/2
  10/1 -> Medelv3/2
  Mux1/1 -> "Inst, Ave"/1
  Medelv/1 -> Pem/1, Mux1/1
  Medelv1/1 -> Pem/2, Mux1/2
  Medelv2/1 -> Pem/3, Mux1/3
  Medelv3/1 -> Pem/4, Mux1/4
  Integral/1 -> 10 seconds/1, 1 minute/1, 30 minutes/1, Medelv/1, Add2/1, Add1/1, Add/1

== system GeneralFEVmodel/Electric Machine model/Subsystem ==
  T : Inport
  w : Inport  Port=2
  Abs2 : Abs
  Constant : Constant  Value=eps
  EM torque1 : Product  Inputs=/*  InputSameDT=on  SaturateOnIntegerOverflow=on  OutDataTypeStr=Inherit: Same as first input
  T*w_ice : Product  Inputs=**  InputSameDT=on  SaturateOnIntegerOverflow=on  OutDataTypeStr=Inherit: Same as first input
  maxP : Saturate  UpperLimit=Pmax  LowerLimit=-Pmax
  maxT : Saturate  UpperLimit=Tmax  LowerLimit=-Tmax
  not div by 0 : Sum  InputSameDT=on  SaturateOnIntegerOverflow=on  OutDataTypeStr=Inherit: Same as first input
  Tlim : Outport  VectorParamsAs1DForOutWhenUnconnected=off
  wires:
  w/1 -> Abs2/1
  T/1 -> T*w_ice/2
  T*w_ice/1 -> maxP/1
  Abs2/1 -> not div by 0/2
  Constant/1 -> not div by 0/1
  maxP/1 -> EM torque1/2
  EM torque1/1 -> maxT/1
  not div by 0/1 -> EM torque1/1, T*w_ice/1
  maxT/1 -> Tlim/1

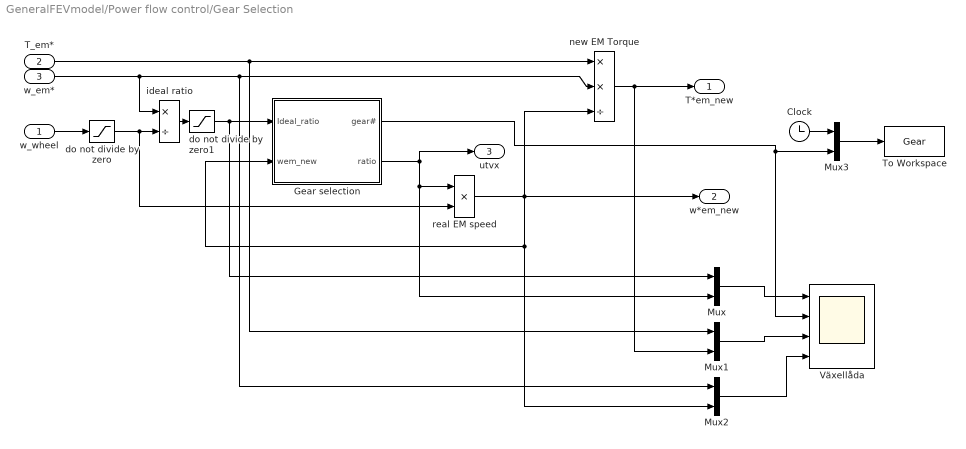
== system GeneralFEVmodel/Power flow control/Gear Selection ==
  w_wheel : Inport
  T_em* : Inport  Port=2
  w_em* : Inport  Port=3
  Clock : Clock
  Gear selection : Subsystem
  Mux{,1..3} (4 alike) : Mux  Inputs=2
  To Workspace : ToWorkspace  VariableName=Gear  SampleTime=-1
  Växellåda : Scope  NumInputPorts=4
  do not divide by zero : Saturate  UpperLimit=inf  LowerLimit=wem_min/utvx_max
  do not divide by zero1 : Saturate  UpperLimit=1.2*max(Utvx_vect)  LowerLimit=eps
  ideal ratio : Product  Inputs=*/  InputSameDT=on  SaturateOnIntegerOverflow=on  OutDataTypeStr=Inherit: Same as first input
  new EM Torque : Product  Inputs=**/  InputSameDT=on  SaturateOnIntegerOverflow=on  OutDataTypeStr=Inherit: Same as first input
  real EM speed : Product  Inputs=**  InputSameDT=on  SaturateOnIntegerOverflow=on  OutDataTypeStr=Inherit: Same as first input
  T*em_new : Outport  VectorParamsAs1DForOutWhenUnconnected=off
  w*em_new : Outport  Port=2  VectorParamsAs1DForOutWhenUnconnected=off
  utvx : Outport  Port=3  VectorParamsAs1DForOutWhenUnconnected=off
  wires:
  w_em*/1 -> ideal ratio/1, Mux2/1, new EM Torque/2
  ideal ratio/1 -> do not divide by zero1/1
  real EM speed/1 -> w*em_new/1, new EM Torque/3, Mux2/2, Gear selection/2(wem_new)
  T_em*/1 -> Mux1/1, new EM Torque/1
  do not divide by zero/1 -> ideal ratio/2, real EM speed/2
  w_wheel/1 -> do not divide by zero/1
  Mux/1 -> Växellåda/1
  Mux1/1 -> Växellåda/3
  Mux2/1 -> Växellåda/4
  Gear selection/2(ratio) -> utvx/1, real EM speed/1, Mux/2
  Gear selection/1(gear#) -> Mux3/2, Växellåda/2
  new EM Torque/1 -> Mux1/2, T*em_new/1
  do not divide by zero1/1 -> Gear selection/1(Ideal_ratio), Mux/1
  Clock/1 -> Mux3/1
  Mux3/1 -> To Workspace/1

== system GeneralFEVmodel/Power flow control/Optimal operating point ==
  Pem* : Inport
  Saturation2 : Saturate  UpperLimit=Pem_max  LowerLimit=-Pem_max
  Saturation3 : Saturate  UpperLimit=Tem_max  LowerLimit=-Tem_max
  Saturation4 : Saturate  UpperLimit=wem_max  LowerLimit=0
  Scope : Scope  NumInputPorts=3
  Topt_em : Lookup  InputValues=PtoTem(:,1)  Table=PtoTem(:,2)  LookUpMeth=Interpolation-Use End Values
  Wopt_em : Lookup  InputValues=PtoTem(:,1)  Table=PtoTem(:,4)  LookUpMeth=Interpolation-Use End Values
  Tem * : Outport  InitialOutput=0  VectorParamsAs1DForOutWhenUnconnected=off
  wem* : Outport  Port=2  InitialOutput=0  VectorParamsAs1DForOutWhenUnconnected=off
  wires:
  Topt_em/1 -> Saturation3/1
  Saturation4/1 -> Scope/3, wem*/1
  Saturation2/1 -> Wopt_em/1, Scope/1, Topt_em/1
  Saturation3/1 -> Scope/2, Tem */1
  Wopt_em/1 -> Saturation4/1
  Pem*/1 -> Saturation2/1

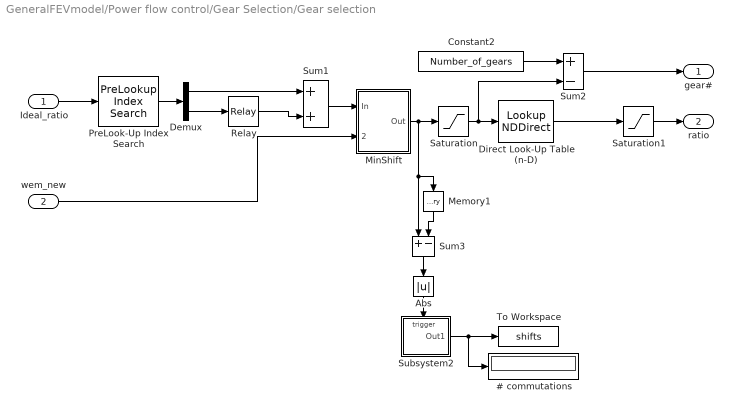
== system GeneralFEVmodel/Power flow control/Gear Selection/Gear selection ==
  Ideal_ratio : Inport
  wem_new : Inport  Port=2
  # commutations : Display
  Abs : Abs
  Constant2 : Constant  Value=Number_of_gears
  Demux : Demux  Outputs=2
      settings: DisplayOption=none
  Direct Look-Up Table (n-D) : LookupNDDirect  NumberOfTableDimensions=1  Table=Utvx_vect
  Memory1 : Memory
  MinShift : Subsystem
  PreLook-Up Index Search : simulink_need_slupdate/PreLookup Index Search  bpData=Utvx_vect  searchMode=Binary Search  cacheBpFlag=off  outputFlag=off  IndexDataType=uint32  extrapMode=Linear Extrapolation  rangeErrorMode=None
      settings: SourceProductBaseCode=SL
  Relay : Relay  OnSwitchValue=0.52  OffSwitchValue=0.48
  Saturation : Saturate  UpperLimit=Number_of_gears-1  LowerLimit=0
  Saturation1 : Saturate  UpperLimit=max(Utvx_vect)  LowerLimit=min(Utvx_vect)
  Subsystem2 : Subsystem  TreatAsAtomicUnit=on
  Sum1 : Sum  SaturateOnIntegerOverflow=on
  Sum2 : Sum  Inputs=+-  SaturateOnIntegerOverflow=on
  Sum3 : Sum  Inputs=+-  SaturateOnIntegerOverflow=on
  To Workspace : ToWorkspace  VariableName=shifts  SampleTime=-1
  gear# : Outport  VectorParamsAs1DForOutWhenUnconnected=off
  ratio : Outport  Port=2  VectorParamsAs1DForOutWhenUnconnected=off
  wires:
  Ideal_ratio/1 -> PreLook-Up Index Search/1
  wem_new/1 -> MinShift/2(Wem_new)
  PreLook-Up Index Search/1 -> Demux/1
  Demux/2 -> Relay/1
  Relay/1 -> Sum1/2
  Direct Look-Up Table (n-D)/1 -> Saturation1/1
  Constant2/1 -> Sum2/1
  Sum2/1 -> gear#/1
  Saturation/1 -> Direct Look-Up Table (n-D)/1, Sum2/2
  Subsystem2/1(Out1) -> # commutations/1, To Workspace/1
  Memory1/1 -> Sum3/2
  Sum3/1 -> Abs/1
  Abs/1 -> Subsystem2/Trigger
  MinShift/1(Out) -> Sum3/1, Memory1/1, Saturation/1
  Sum1/1 -> MinShift/1(In)
  Saturation1/1 -> ratio/1
  Demux/1 -> Sum1/1

== system GeneralFEVmodel/Power flow control/Gear Selection/Gear selection/MinShift ==
  In : Inport
  Wem_new : Inport  Port=2
  Abs1 : Abs
  Memory2 : Memory
  Memory4 : Memory
  Pulse Generator : DiscretePulseGenerator  Period=4  PulseWidth=2  SampleTime=0.1
  Scope1 : Scope
  Subsystem : Subsystem
  Sum4 : Sum  Inputs=+++  SaturateOnIntegerOverflow=on
  Sum5 : Sum  Inputs=+-  SaturateOnIntegerOverflow=on
  w<xx : Relay  OnSwitchValue=wem_min*1.2  OffSwitchValue=wem_min*1.1  OnOutputValue=0  OffOutputValue=1
  w>yy : Relay  OnSwitchValue=wem_max*0.66  OffSwitchValue=wem_max*0.65
  Out : Outport  VectorParamsAs1DForOutWhenUnconnected=off
  wires:
  w>yy/1 -> Sum4/2
  w<xx/1 -> Sum4/3
  Pulse Generator/1 -> Scope1/1, Sum4/1
  Memory2/1 -> Sum5/2
  Sum5/1 -> Abs1/1
  Wem_new/1 -> w>yy/1, w<xx/1
  In/1 -> Subsystem/1(In1)
  Subsystem/1(Out1) -> Out/1
  Memory4/1 -> Sum5/1, Memory2/1
  Sum4/1 -> Memory4/1
  Abs1/1 -> Subsystem/Trigger

== system GeneralFEVmodel/Power flow control/Gear Selection/Gear selection/Subsystem2 ==
  Trigger : TriggerPort  TriggerType=either  VariantControl=Variant
  Constant : Constant
  Memory : Memory  InheritSampleTime=on
  Sum : Sum  InputSameDT=on  SaturateOnIntegerOverflow=on  OutDataTypeStr=Inherit: Same as first input
  Out1 : Outport  VectorParamsAs1DForOutWhenUnconnected=off
  wires:
  Sum/1 -> Memory/1, Out1/1
  Memory/1 -> Sum/2
  Constant/1 -> Sum/1

== system GeneralFEVmodel/Power flow control/Gear Selection/Gear selection/MinShift/Subsystem ==
  In1 : Inport
  Trigger : TriggerPort  TriggerType=either  VariantControl=Variant
  Zero-Order Hold : ZeroOrderHold  SampleTime=-1
  Out1 : Outport
  wires:
  In1/1 -> Zero-Order Hold/1
  Zero-Order Hold/1 -> Out1/1
